simulink model "cruiseControlRBTCovExample"  (R2022b)
settings: Solver=FixedStepDiscrete  StartTime=0.0  StopTime=10.0  FixedStep=0.01  RelTol=1e-3  EnableMultiTasking=on
undefined symbols (not defined in the file): DiscIntNeverNeededParam
settings Model: Creator=The MathWorks, Inc.  LastModifiedBy=The MathWorks, Inc.
settings SolverCC: AlgebraicLoopSolver=TrustRegion  MaxZcPerStep=1
settings DataIOCC: LimitDataPoints=on  SaveFormat=Array  ReturnWorkspaceOutputs=off
settings OptimizationCC: ConditionallyExecuteInputs=off  DefaultParameterBehavior=Inlined  InlineInvariantSignals=on  ExpressionDepthLimit=2147483647  InitFltsAndDblsToZero=on  EfficientMapNaN2IntZero=off  LifeSpan=inf
settings DebuggingCC: SaveWithParameterizedLinksMsg=none  UnderspecifiedInitializationDetection=Classic  MergeDetectMultiDrivingBlocksExec=none  SignalResolutionControl=TryResolveAllWithWarning  SolverPrmCheckMsg=warning  FcnCallInpInsideContextMsg=warning  UnconnectedInputMsg=warning  UnconnectedOutputMsg=warning  UnconnectedLineMsg=warning  AllowSymbolicDim=off  StateNameClashWarn=warning  SFUnexpectedBacktrackingDiag=warning  SFNoUnconditionalDefaultTransitionDiag=warning  SFExecutionAtInitializationDiag=none  SFMachineParentedDataDiag=warning  ArithmeticOperatorsInVariantConditions=warning
settings HardwareCC: ProdBitPerPointer=32  ProdBitPerSizeT=32  ProdBitPerPtrDiffT=32  ProdLargestAtomicFloat=None  ProdIntDivRoundTo=Undefined  ProdEndianess=Unspecified  ProdWordSize=32  ProdHWDeviceType=32-bit Generic
settings ModelReferenceCC: EnableRefExpFcnMdlSchedulingChecks=on  PropagateSignalLabelsOutOfModel=off
settings SFSimCC: SimUseLocalCustomCode=off  CustomCodeUndefinedFunction=UseInterfaceOnly
settings RTWCC: RTWUseLocalCustomCode=off  DLArmComputeVersion=19.05
settings CodeAppCC: StateflowObjectComments=on
settings GRTTargetCC: TargetFcnLib=ansi_tfl_tmw.mat  TargetLangStandard=C89/C90 (ANSI)  CombineOutputUpdateFcns=off  GRTInterface=on
settings ConfigComp: CovMetricSettings=dcme  CovHTMLOptions=-sRT=1 -sVT=0 -aTS=1 -agT=1 -bRG=1 -bTC=1 -hTR=0 -nFC=0 -nFD=0 -scm=1 -bcm=1 -xEv=0 -xEM=0 -req=1  DVMakeOutputFilesUnique=off  DVParameterConfiguration=UseParameterConfigFile  DVParameters=on  DVModelCoverageObjectives=MCDC  DVMaxTestCaseSteps=500  DVTestSuiteOptimization=Auto  DVAssertions=EnableAll  DVProofAssumptions=EnableAll  DVDetectActiveLogic=on  DVProvingStrategy=FindViolation  DVReduceRationalApprox=off  DVRebuildModelRepresentation=Always

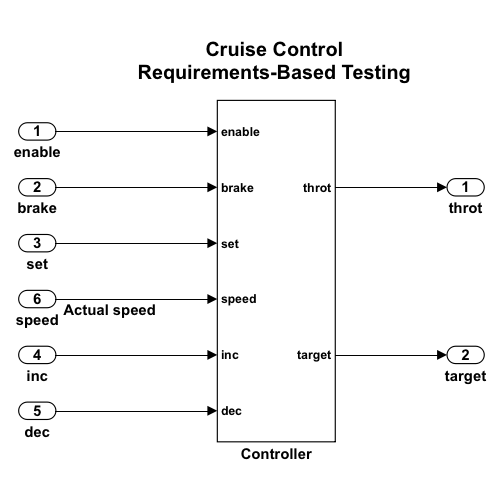
[thumbnail: Simulink's stored preview of the top-level diagram]
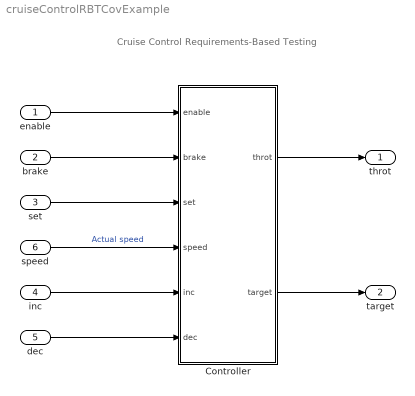
== system cruiseControlRBTCovExample ==
  note: Cruise Control
      | Requirements-Based Testing
  enable : Inport  OutDataTypeStr=boolean
  brake : Inport  Port=2  OutDataTypeStr=boolean
  set : Inport  Port=3  OutDataTypeStr=boolean
  inc : Inport  Port=4  OutDataTypeStr=boolean
  dec : Inport  Port=5  OutDataTypeStr=boolean
  speed : Inport  Port=6  OutDataTypeStr=double
  Controller : Subsystem
  throt : Outport  VectorParamsAs1DForOutWhenUnconnected=off
  target : Outport  Port=2  VectorParamsAs1DForOutWhenUnconnected=off
  wires:
  enable/1 -> Controller/1(enable)
  brake/1 -> Controller/2(brake)
  set/1 -> Controller/3(set)
  Controller/1(throt) -> throt/1
  inc/1 -> Controller/5(inc)
  dec/1 -> Controller/6(dec)
  Controller/2(target) -> target/1
  speed/1 -> Controller/4(speed)  "Actual speed"

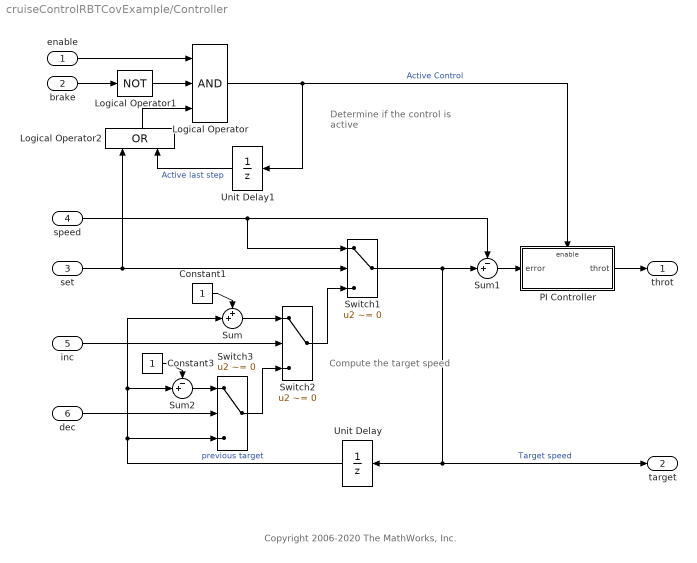
== system cruiseControlRBTCovExample/Controller ==
  note: Copyright 2006-2020 The MathWorks, Inc.
  note: Determine if the
      | control is active
  note: Compute the
      | target speed
  enable : Inport  OutDataTypeStr=boolean
  brake : Inport  Port=2  OutDataTypeStr=boolean
  set : Inport  Port=3  OutDataTypeStr=boolean
  speed : Inport  Port=4  OutDataTypeStr=double
  inc : Inport  Port=5  OutDataTypeStr=boolean
  dec : Inport  Port=6  OutDataTypeStr=boolean
  Constant1 : Constant
  Constant3 : Constant
  Logical Operator : Logic  Inputs=3  AllPortsSameDT=off  OutDataTypeStr=boolean
  Logical Operator1 : Logic  Operator=NOT  AllPortsSameDT=off  OutDataTypeStr=boolean
  Logical Operator2 : Logic  Operator=OR  AllPortsSameDT=off  OutDataTypeStr=boolean
  PI Controller : Subsystem
  Sum : Sum  Inputs=++|
  Sum1 : Sum  Inputs=-+|
  Sum2 : Sum  Inputs=-+|
  Switch1 : Switch  Criteria=u2 ~= 0  SaturateOnIntegerOverflow=off  InputSameDT=off
  Switch2 : Switch  Criteria=u2 ~= 0  SaturateOnIntegerOverflow=off  InputSameDT=off
  Switch3 : Switch  Criteria=u2 ~= 0  SaturateOnIntegerOverflow=off  InputSameDT=off
  Unit Delay : UnitDelay  SampleTime=0.01  HasFrameUpgradeWarning=on
  Unit Delay1 : UnitDelay  SampleTime=0.01  HasFrameUpgradeWarning=on
  throt : Outport  VectorParamsAs1DForOutWhenUnconnected=off
  target : Outport  Port=2  VectorParamsAs1DForOutWhenUnconnected=off
  wires:
  brake/1 -> Logical Operator1/1
  enable/1 -> Logical Operator/1
  Logical Operator1/1 -> Logical Operator/2
  set/1 -> Switch1/2, Logical Operator2/1
  speed/1 -> Sum1/1, Switch1/1
  inc/1 -> Switch2/2
  Constant1/1 -> Sum/1
  Sum/1 -> Switch2/1
  dec/1 -> Switch3/2
  Constant3/1 -> Sum2/1
  Sum2/1 -> Switch3/1
  Switch2/1 -> Switch1/3
  Switch3/1 -> Switch2/3
  Unit Delay/1 -> Sum/2, Sum2/2, Switch3/3  "previous target"
  Switch1/1 -> Unit Delay/1, target/1, Sum1/2  "Target speed"
  Logical Operator2/1 -> Logical Operator/3
  Unit Delay1/1 -> Logical Operator2/2  "Active last step"
  Logical Operator/1 -> Unit Delay1/1, PI Controller/Enable  "Active Control"
  Sum1/1 -> PI Controller/1(error)
  PI Controller/1(throt) -> throt/1

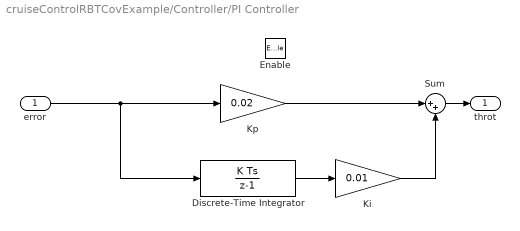
== system cruiseControlRBTCovExample/Controller/PI Controller ==
  error : Inport
  Enable : EnablePort
  Discrete-Time Integrator : DiscreteIntegrator  SampleTime=0.01  LimitOutput=on  UpperSaturationLimit=5  LowerSaturationLimit=-5  ICPrevOutput=DiscIntNeverNeededParam  ICPrevScaledInput=DiscIntNeverNeededParam
  Ki : Gain  Gain=0.01
  Kp : Gain  Gain=0.02
  Sum : Sum  Inputs=|++
  throt : Outport  VectorParamsAs1DForOutWhenUnconnected=off
  wires:
  Kp/1 -> Sum/1
  Ki/1 -> Sum/2
  Discrete-Time Integrator/1 -> Ki/1
  error/1 -> Kp/1, Discrete-Time Integrator/1
  Sum/1 -> throt/1
